simulink model "CommandePWM"  (R2022a)
settings: Solver=FixedStepAuto  StartTime=0.0  StopTime=inf  RelTol=1e-3  EnableMultiTasking=on
libraries: arduinolib x2, simulink x1
settings Model: ExtModeTrigDuration=2  Creator=xpess  LastModifiedBy=xavier.pessoles2
settings OptimizationCC: EnhancedBackFolding=on  PassReuseOutputArgsAs=Individual arguments  ZeroExternalMemoryAtStartup=off  ZeroInternalMemoryAtStartup=off  MaxStackSize=64  OptimizeBlockOrder=speed  DifferentSizesBufferReuse=on  OptimizationCustomize=off  EfficientTunableParamExpr=on
settings DebuggingCC: ParameterTunabilityLossMsg=error  UnconnectedInputMsg=warning  UnconnectedOutputMsg=warning  UnconnectedLineMsg=warning
settings HardwareCC: ProdBitPerPointer=32  ProdBitPerSizeT=32  ProdBitPerPtrDiffT=32  ProdLargestAtomicInteger=Long  ProdLargestAtomicFloat=Double  ProdWordSize=32  ProdHWDeviceType=ARM Compatible->ARM Cortex
settings SFSimCC: MATLABDynamicMemAlloc=off
settings RTWCC: SystemTargetFile=ert.tlc  HardwareBoard=Arduino Due  TemplateMakefile=ert_default_tmf  Toolchain=Arduino ARM  BuildConfiguration=Faster Runs  DLArmComputeVersion=19.05
settings CodeAppCC: ForceParamTrailComments=on  IgnoreCustomStorageClasses=off  OperatorAnnotations=on  SimulinkDataObjDesc=on  SFDataObjDesc=on  InsertBlockDesc=on
settings ERTTargetCC: SupportContinuousTime=on  SupportVariableSizeSignals=on  ExtModeTransport=3  ExtModeStaticAlloc=on  ExtModeStaticAllocSize=24576  ExtModeMexFile=ext_xcp  ExtModeIntrfLevel=Level2 - Open

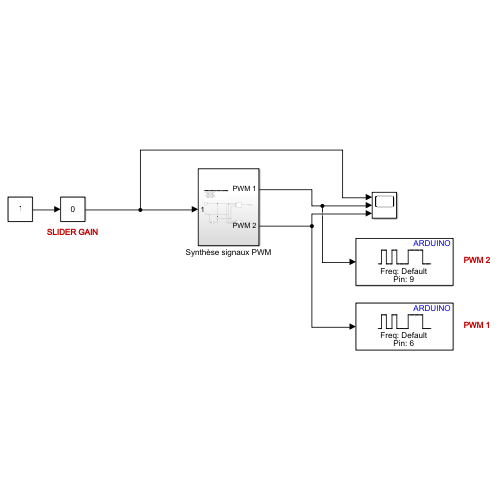
[thumbnail: Simulink's stored preview of the top-level diagram]
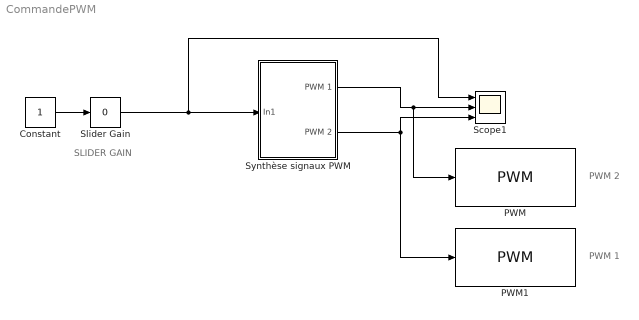
== system CommandePWM ==
  note: SLIDER GAIN
  note: PWM 2
  note: PWM 1
  Constant : Constant
  PWM : arduinolib/PWM  pinNumber=9  frequencyType=Default  desiredFrequency=490.2  achievableFrequency=490.2
  PWM1 : arduinolib/PWM  pinNumber=6  frequencyType=Default  desiredFrequency=490.2  achievableFrequency=490.2
  Scope1 : Scope  NumInputPorts=3
  Slider Gain : simulink/Math Operations/Slider Gain  gain=0  low=-255  high=255
  Synthèse signaux PWM : Subsystem
  wires:
  Slider Gain/1 -> Scope1/1, Synthèse signaux PWM/1(In1)
  Synthèse signaux PWM/1(PWM 1) -> PWM/1, Scope1/2
  Synthèse signaux PWM/2(PWM 2) -> PWM1/1, Scope1/3
  Constant/1 -> Slider Gain/1

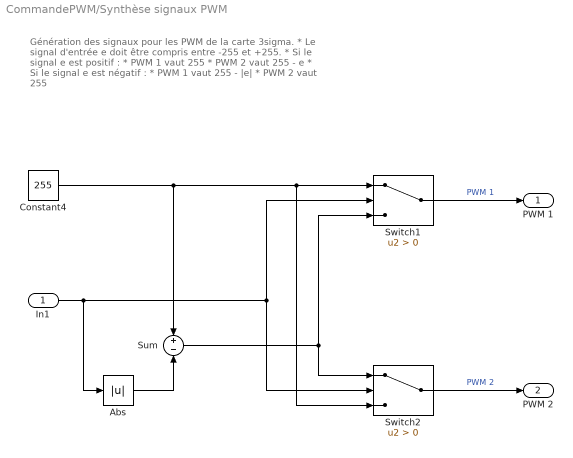
== system CommandePWM/Synthèse signaux PWM ==
  note: Génération des signaux pour les PWM de la carte 3sigma.
      | * Le signal d'entrée e doit être compris entre -255 et +255.
      | * Si le signal e est positif :
      | * PWM 1 vaut 255
      | * PWM 2 vaut 255 - e
      | * Si le signal e est négatif :
      | * PWM 1 vaut 255 - |e|
      | * PWM 2 vaut 255
  In1 : Inport
  Abs : Abs  SaturateOnIntegerOverflow=off
  Constant4 : Constant  Value=255
  Sum : Sum  Inputs=+|-
  Switch1 : Switch  Criteria=u2 > Threshold  SaturateOnIntegerOverflow=off  InputSameDT=off
  Switch2 : Switch  Criteria=u2 > Threshold  SaturateOnIntegerOverflow=off  InputSameDT=off
  PWM 1 : Outport
  PWM 2 : Outport  Port=2
  wires:
  Constant4/1 -> Sum/1, Switch2/3, Switch1/1
  Abs/1 -> Sum/2
  Switch1/1 -> PWM 1/1  "PWM 1"
  In1/1 -> Switch1/2, Switch2/2, Abs/1
  Switch2/1 -> PWM 2/1  "PWM 2"
  Sum/1 -> Switch1/3, Switch2/1
